simulink model "MBD_Week2_Prob1"  (R2020a)
settings: Solver=VariableStepAuto  StartTime=0.0  StopTime=inf  RelTol=1e-3
settings Model: Creator=Noel Varghese  LastModifiedBy=Noel Varghese

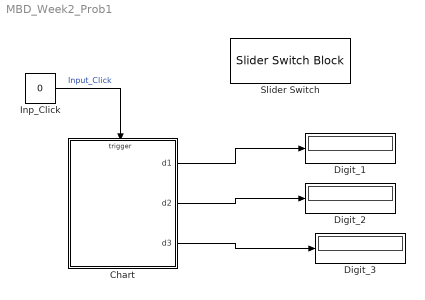
== system MBD_Week2_Prob1 ==
  Chart : Stateflow chart  TreatAsAtomicUnit=on
  Digit_1 : Display
  Digit_2 : Display
  Digit_3 : Display
  Inp_Click : Constant  Value=0
  Slider Switch : SliderSwitchBlock
      settings: Values={{'Off', 'On'}, [0 1]}
  wires:
  Inp_Click/1 -> Chart/Trigger  "Input_Click"
  Chart/1(d1) -> Digit_1/1
  Chart/2(d2) -> Digit_2/1
  Chart/3(d3) -> Digit_3/1

== stateflow chart MBD_Week2_Prob1/Chart ==
  state Digit_1 [parallel]
    settings: executionOrder=1
    state One
      en: d1=1;
    state Two
      en: d1=2;
    state Zero
      en: d1=0;
    state Three
      en: d1=3;
    state Four
      en: d1=4;
    (default) -> Digit_1.Zero
    Digit_1.Two -> Digit_1.Three : InpClick
    Digit_1.Zero -> Digit_1.One : InpClick
    Digit_1.One -> Digit_1.Two : InpClick
    Digit_1.Four -> Digit_1.Zero : InpClick/{Digit_2.Inc2;}
    Digit_1.Three -> Digit_1.Four : InpClick
  state Digit_2 [parallel]
    settings: executionOrder=2
    state One
      en: d2=1;
    state Two
      en: d2=2;
    state Zero
      en: d2=0;
    state Three
      en: d2=3;
    state Four
      en: d2=4;
    (default) -> Digit_2.Zero
    Digit_2.Two -> Digit_2.Three : Inc2
    Digit_2.Zero -> Digit_2.One : Inc2
    Digit_2.One -> Digit_2.Two : Inc2
    Digit_2.Four -> Digit_2.Zero : Inc2/{Digit_3.Inc3;}
    Digit_2.Three -> Digit_2.Four : Inc2
  state Digit_3 [parallel]
    settings: executionOrder=3
    state One
      en: d3=1;
    state Two
      en: d3=2;
    state Zero
      en: d3=0;
    state Three
      en: d3=3;
    state Four
      en: d3=4;
    (default) -> Digit_3.Zero
    Digit_3.Two -> Digit_3.Three : Inc3
    Digit_3.Zero -> Digit_3.One : Inc3
    Digit_3.One -> Digit_3.Two : Inc3
    Digit_3.Four -> Digit_3.Zero : Inc3
    Digit_3.Three -> Digit_3.Four : Inc3
  data: d1 output; d2 output; d3 output
  events: Inc2 local FUNCTION_CALL_EVENT; Inc3 local FUNCTION_CALL_EVENT; InpClick input EITHER_EDGE_EVENT
